simulink model "pendulum3D_nonlinear_control_cascade_simulation"  (R2017a)
settings: Solver=FixedStepAuto  StartTime=0.0  StopTime=30  FixedStep=dt  RelTol=1e-3
values from neighbouring files (symbols this model uses):
  d_x = 7    [simulation_initalization.m]
  d_y = 4    [simulation_initalization.m]
  dt = 1e-3    (= 0.001)    [f_simulink3d.m]    (also in simulation_initalization.m)
  Kdx_t = 3.324    [simulation_initalization.m]
  Kdy_t = 0.4079    [simulation_initalization.m]
  Kix = 0.103    [simulation_initalization.m]
  Kiy = 0.07209    [simulation_initalization.m]
  Kpx = 0.577    [simulation_initalization.m]
  Kpx_t = 4.786    [simulation_initalization.m]
  Kpy = 0.7879    [simulation_initalization.m]
  Kpy_t = 1.002    [simulation_initalization.m]
  L = 2.0    (= 2)    [compensator_phix.m]    (also in compensator_phiy.m; f_simulink3d.m; pendulum_dynamics.m; simulation_initalization.m)
  phi_init = [phix_init, phiy_init]    [simulation_initalization.m]
  pt_init = [x_init, y_init, z_init]    [simulation_initalization.m]
  x_init = 2.6192    [simulation_initalization.m]
  y_init = 0    [simulation_initalization.m]
  z_init = 2.24    [simulation_initalization.m]
libraries: simulink x4, sharedTrackingLibrary x1
settings Model: Creator=Workstation  LastModifiedBy=Jan

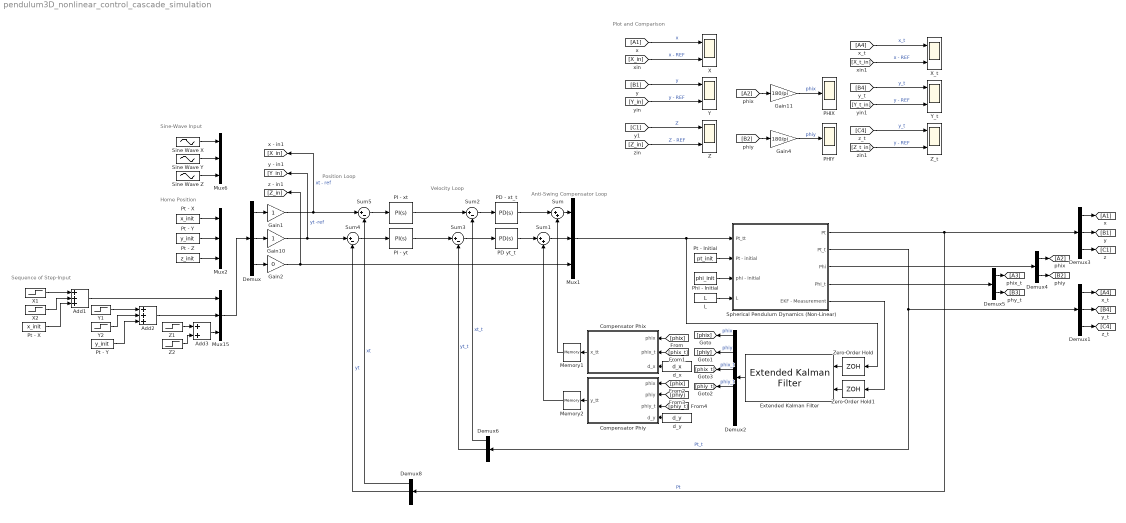
== system pendulum3D_nonlinear_control_cascade_simulation ==
  note: Sequence of Step-Input
  note: Home Position
  note: Sine-Wave Input
  note: Position Loop
  note: Velocity Loop
  note: Anti-Swing Compensator Loop
  note: Plot and Comparison
  Add1 : Sum  Inputs=+++
  Add2 : Sum  Inputs=+++
  Add3 : Sum
  Compensator Phix : MATLAB Function  TreatAsAtomicUnit=on
  Compensator Phiy : MATLAB Function  TreatAsAtomicUnit=on
  Demux{,1,3,6,8} (5 alike) : Demux  Outputs=3
  Demux2 : Demux  Outputs=6
  Demux4 : Demux  Outputs=2
  Demux5 : Demux  Outputs=2
  Extended Kalman Filter : sharedTrackingLibrary/Extended Kalman Filter  StateTransitionFcn=f_simulink3d  HasStateTransitionJacobianFcn=off  HasAdditiveProcessNoise=Additive  ProcessNoise=Q  HasTimeVaryingProcessNoise=off  HasStateTransitionFcnExtraArgument=1  InitialState=zeros(6,1)  InitialStateCovariance=P  MeasurementFcn1=h_simulink3d  HasMeasurementJacobianFcn1=off  HasMeasurementEnablePort1=off  HasAdditiveMeasurementNoise1=Additive  MeasurementNoise1=R  HasTimeVaryingMeasurementNoise1=off  HasMeasurementFcnExtraArgument1=0  MeasurementFcn2=myMeasurementFcn  HasMeasurementJacobianFcn2=off  HasMeasurementEnablePort2=off  HasAdditiveMeasurementNoise2=Additive  MeasurementNoise2=1  HasTimeVaryingMeasurementNoise2=off  HasMeasurementFcnExtraArgument2=0  MeasurementFcn3=myMeasurementFcn  HasMeasurementJacobianFcn3=off  HasMeasurementEnablePort3=off  HasAdditiveMeasurementNoise3=Additive  MeasurementNoise3=1  HasTimeVaryingMeasurementNoise3=off  HasMeasurementFcnExtraArgument3=0  MeasurementFcn4=myMeasurementFcn  HasMeasurementJacobianFcn4=off  HasMeasurementEnablePort4=off  HasAdditiveMeasurementNoise4=Additive  MeasurementNoise4=1  HasTimeVaryingMeasurementNoise4=off  HasMeasurementFcnExtraArgument4=0  MeasurementFcn5=myMeasurementFcn  HasMeasurementJacobianFcn5=off  HasMeasurementEnablePort5=off  HasAdditiveMeasurementNoise5=Additive  MeasurementNoise5=1  HasTimeVaryingMeasurementNoise5=off  HasMeasurementFcnExtraArgument5=0  EnableMultirate=off  StateTransitionFcnSampleTime=1  MeasurementFcn1SampleTime=1  MeasurementFcn2SampleTime=1  MeasurementFcn3SampleTime=1  MeasurementFcn4SampleTime=1  MeasurementFcn5SampleTime=1  UseCurrentEstimator=on  OutputStateCovariance=off  DataType=double  SampleTime=dt  NumberOfMeasurements=1
  Gain1 : Gain
  Gain10 : Gain
  Gain11 : Gain  Gain=180/pi
  Gain2 : Gain  Gain=0
  Gain4 : Gain  Gain=180/pi
  L : Constant  Value=L
  Memory1 : Memory
  Memory2 : Memory
  Mux{1..2,6,15} (4 alike) : Mux  Inputs=3
  PD - xt_t : simulink/Continuous/PID Controller  Controller=PD  TimeDomain=Continuous-time  SampleTime=-1  IntegratorMethod=Forward Euler  FilterMethod=Forward Euler  Form=Parallel  UseFilter=on  ControllerParametersSource=internal  P=Kpx_t  I=1  D=Kdx_t  N=100  InitialConditionSource=internal  InitialConditionForIntegrator=0  InitialConditionForFilter=0  ExternalReset=none  LimitOutput=off  UpperSaturationLimit=inf  LowerSaturationLimit=-inf  LinearizeAsGain=on  AntiWindupMode=none  Kb=1  TrackingMode=off  Kt=1  PParamMin=[]  PParamMax=[]  IParamMin=[]  IParamMax=[]  DParamMin=[]  DParamMax=[]  NParamMin=[]  NParamMax=[]  KbParamMin=[]  KbParamMax=[]  KtParamMin=[]  KtParamMax=[]  POutMin=[]  POutMax=[]  IOutMin=[]  IOutMax=[]  DOutMin=[]  DOutMax=[]  NOutMin=[]  NOutMax=[]  KbOutMin=[]  KbOutMax=[]  KtOutMin=[]  KtOutMax=[]  IntegratorOutMin=[]  IntegratorOutMax=[]  FilterOutMin=[]  FilterOutMax=[]  SumOutMin=[]  SumOutMax=[]  SumI1OutMin=[]  SumI1OutMax=[]  SumI2OutMin=[]  SumI2OutMax=[]  SumI3OutMin=[]  SumI3OutMax=[]  SumDOutMin=[]  SumDOutMax=[]  SaturationOutMin=[]  SaturationOutMax=[]  IntegratorContinuousStateAttributes=''  IntegratorStateMustResolveToSignalObject=off  IntegratorRTWStateStorageClass=Auto  FilterContinuousStateAttributes=''  FilterStateMustResolveToSignalObject=off  FilterRTWStateStorageClass=Auto  DifferentiatorICPrevScaledInput=0  DifferentiatorOutMin=[]  DifferentiatorOutMax=[]  InitialConditionSetting=State (most efficient)
  PD yt_t : simulink/Continuous/PID Controller  Controller=PD  TimeDomain=Continuous-time  SampleTime=-1  IntegratorMethod=Forward Euler  FilterMethod=Forward Euler  Form=Parallel  UseFilter=on  ControllerParametersSource=internal  P=Kpy_t  I=1  D=Kdy_t  N=100  InitialConditionSource=internal  InitialConditionForIntegrator=0  InitialConditionForFilter=0  ExternalReset=none  LimitOutput=off  UpperSaturationLimit=inf  LowerSaturationLimit=-inf  LinearizeAsGain=on  AntiWindupMode=none  Kb=1  TrackingMode=off  Kt=1  PParamMin=[]  PParamMax=[]  IParamMin=[]  IParamMax=[]  DParamMin=[]  DParamMax=[]  NParamMin=[]  NParamMax=[]  KbParamMin=[]  KbParamMax=[]  KtParamMin=[]  KtParamMax=[]  POutMin=[]  POutMax=[]  IOutMin=[]  IOutMax=[]  DOutMin=[]  DOutMax=[]  NOutMin=[]  NOutMax=[]  KbOutMin=[]  KbOutMax=[]  KtOutMin=[]  KtOutMax=[]  IntegratorOutMin=[]  IntegratorOutMax=[]  FilterOutMin=[]  FilterOutMax=[]  SumOutMin=[]  SumOutMax=[]  SumI1OutMin=[]  SumI1OutMax=[]  SumI2OutMin=[]  SumI2OutMax=[]  SumI3OutMin=[]  SumI3OutMax=[]  SumDOutMin=[]  SumDOutMax=[]  SaturationOutMin=[]  SaturationOutMax=[]  IntegratorContinuousStateAttributes=''  IntegratorStateMustResolveToSignalObject=off  IntegratorRTWStateStorageClass=Auto  FilterContinuousStateAttributes=''  FilterStateMustResolveToSignalObject=off  FilterRTWStateStorageClass=Auto  DifferentiatorICPrevScaledInput=0  DifferentiatorOutMin=[]  DifferentiatorOutMax=[]  InitialConditionSetting=State (most efficient)
  PHIX : Scope
  PHIY : Scope
  PI - xt : simulink/Continuous/PID Controller  Controller=PI  TimeDomain=Continuous-time  SampleTime=-1  IntegratorMethod=Forward Euler  FilterMethod=Forward Euler  Form=Parallel  UseFilter=on  ControllerParametersSource=internal  P=Kpx  I=Kix  D=Kix  N=100  InitialConditionSource=internal  InitialConditionForIntegrator=0  InitialConditionForFilter=0  ExternalReset=none  LimitOutput=off  UpperSaturationLimit=inf  LowerSaturationLimit=-inf  LinearizeAsGain=on  AntiWindupMode=none  Kb=1  TrackingMode=off  Kt=1  PParamMin=[]  PParamMax=[]  IParamMin=[]  IParamMax=[]  DParamMin=[]  DParamMax=[]  NParamMin=[]  NParamMax=[]  KbParamMin=[]  KbParamMax=[]  KtParamMin=[]  KtParamMax=[]  POutMin=[]  POutMax=[]  IOutMin=[]  IOutMax=[]  DOutMin=[]  DOutMax=[]  NOutMin=[]  NOutMax=[]  KbOutMin=[]  KbOutMax=[]  KtOutMin=[]  KtOutMax=[]  IntegratorOutMin=[]  IntegratorOutMax=[]  FilterOutMin=[]  FilterOutMax=[]  SumOutMin=[]  SumOutMax=[]  SumI1OutMin=[]  SumI1OutMax=[]  SumI2OutMin=[]  SumI2OutMax=[]  SumI3OutMin=[]  SumI3OutMax=[]  SumDOutMin=[]  SumDOutMax=[]  SaturationOutMin=[]  SaturationOutMax=[]  IntegratorContinuousStateAttributes=''  IntegratorStateMustResolveToSignalObject=off  IntegratorRTWStateStorageClass=Auto  FilterContinuousStateAttributes=''  FilterStateMustResolveToSignalObject=off  FilterRTWStateStorageClass=Auto  DifferentiatorICPrevScaledInput=0  DifferentiatorOutMin=[]  DifferentiatorOutMax=[]  InitialConditionSetting=State (most efficient)
  PI - yt : simulink/Continuous/PID Controller  Controller=PI  TimeDomain=Continuous-time  SampleTime=-1  IntegratorMethod=Forward Euler  FilterMethod=Forward Euler  Form=Parallel  UseFilter=on  ControllerParametersSource=internal  P=Kpy  I=Kiy  D=0  N=100  InitialConditionSource=internal  InitialConditionForIntegrator=0  InitialConditionForFilter=0  ExternalReset=none  LimitOutput=off  UpperSaturationLimit=inf  LowerSaturationLimit=-inf  LinearizeAsGain=on  AntiWindupMode=none  Kb=1  TrackingMode=off  Kt=1  PParamMin=[]  PParamMax=[]  IParamMin=[]  IParamMax=[]  DParamMin=[]  DParamMax=[]  NParamMin=[]  NParamMax=[]  KbParamMin=[]  KbParamMax=[]  KtParamMin=[]  KtParamMax=[]  POutMin=[]  POutMax=[]  IOutMin=[]  IOutMax=[]  DOutMin=[]  DOutMax=[]  NOutMin=[]  NOutMax=[]  KbOutMin=[]  KbOutMax=[]  KtOutMin=[]  KtOutMax=[]  IntegratorOutMin=[]  IntegratorOutMax=[]  FilterOutMin=[]  FilterOutMax=[]  SumOutMin=[]  SumOutMax=[]  SumI1OutMin=[]  SumI1OutMax=[]  SumI2OutMin=[]  SumI2OutMax=[]  SumI3OutMin=[]  SumI3OutMax=[]  SumDOutMin=[]  SumDOutMax=[]  SaturationOutMin=[]  SaturationOutMax=[]  IntegratorContinuousStateAttributes=''  IntegratorStateMustResolveToSignalObject=off  IntegratorRTWStateStorageClass=Auto  FilterContinuousStateAttributes=''  FilterStateMustResolveToSignalObject=off  FilterRTWStateStorageClass=Auto  DifferentiatorICPrevScaledInput=0  DifferentiatorOutMin=[]  DifferentiatorOutMax=[]  InitialConditionSetting=State (most efficient)
  Phi - Initial : Constant  Value=phi_init
  Pt - Initial : Constant  Value=pt_init
  Pt - X : Constant  Value=x_init
  "Pt - X " : Constant  Value=x_init
  Pt - Y : Constant  Value=y_init
  "Pt - Y " : Constant  Value=y_init
  Pt - Z : Constant  Value=z_init
  Sine Wave X : Sin  Amplitude=0.5  Bias=x_init  Frequency=2*pi*0.07  SampleTime=0
  Sine Wave Y : Sin  Amplitude=0.3  Bias=y_init  Frequency=2*pi*0.09  SampleTime=0
  Sine Wave Z : Sin  Amplitude=0.25  Bias=z_init  Frequency=2*pi*0.15  SampleTime=0
  Spherical Pendulum Dynamics (Non-Linear) : Subsystem
  Sum : Sum  Inputs=|++
  Sum1 : Sum  Inputs=|++
  Sum{2..5} (4 alike) : Sum  Inputs=|+-
  X : Scope  NumInputPorts=2
  X1 : Step  After=0.4  SampleTime=0
  X2 : Step  Time=10  After=-0.8  SampleTime=0
  X_t : Scope  NumInputPorts=2
  Y : Scope  NumInputPorts=2
  Y1 : Step  Time=2  After=0.4  SampleTime=0
  Y2 : Step  Time=13  After=-0.8  SampleTime=0
  Y_t : Scope  NumInputPorts=2
  Z : Scope  NumInputPorts=2
  Z1 : Step  Time=3  After=0.4  SampleTime=0
  Z2 : Step  Time=9  After=-0.2  SampleTime=0
  Z_t : Scope  NumInputPorts=2
  Zero-Order Hold : ZeroOrderHold  SampleTime=dt
  Zero-Order Hold1 : ZeroOrderHold  SampleTime=dt
  d_x : Constant  Value=d_x
  d_y : Constant  Value=d_y
  wires:
  Zero-Order Hold/1 -> Extended Kalman Filter/1
  Zero-Order Hold1/1 -> Extended Kalman Filter/2
  Spherical Pendulum Dynamics (Non-Linear)/5(EKF - Measurement) -> Zero-Order Hold1/1
  Extended Kalman Filter/1 -> Demux2/1
  Sum1/1 -> Mux1/2
  PD - xt_t/1 -> Sum/1
  Sum/1 -> Mux1/1
  Mux1/1 -> Zero-Order Hold/1, Spherical Pendulum Dynamics (Non-Linear)/1(Pt_tt)
  Pt - Initial/1 -> Spherical Pendulum Dynamics (Non-Linear)/2(Pt - initial)
  Phi - Initial/1 -> Spherical Pendulum Dynamics (Non-Linear)/3(phi - initial)
  Demux5/1 -> [A3]
  Spherical Pendulum Dynamics (Non-Linear)/3(Phi) -> Demux4/1
  Demux5/2 -> [B3]
  Demux4/2 -> [B2]
  Spherical Pendulum Dynamics (Non-Linear)/4(Phi_t) -> Demux5/1
  Demux4/1 -> [A2]
  Demux3/2 -> [B1]
  Demux3/1 -> [A1]
  Spherical Pendulum Dynamics (Non-Linear)/1(Pt) -> Demux8/1, Demux3/1  "Pt"
  Demux3/3 -> [C1]
  Demux1/2 -> [B4]
  Demux1/3 -> [C4]
  [C1] -> Z/1  "Z"
  [Y_in] -> Y/2  "y - REF"
  [Z_in] -> Z/2  "Z - REF"
  Gain11/1 -> PHIX/1  "phix"
  [B2] -> Gain4/1
  Gain4/1 -> PHIY/1  "phiy"
  [A1] -> X/1  "x"
  [B1] -> Y/1  "y"
  [A2] -> Gain11/1
  [X_in] -> X/2  "x - REF"
  [B4] -> Y_t/1  "y_t"
  [A4] -> X_t/1  "x_t"
  [Z_t_in] -> Z_t/2  "y - REF"
  [X_t_in] -> X_t/2  "x - REF"
  [Y_t_in] -> Y_t/2  "y - REF"
  [C4] -> Z_t/1  "y_t"
  Sum2/1 -> PD - xt_t/1
  PD yt_t/1 -> Sum1/1
  Sum4/1 -> PI - yt/1
  Sum5/1 -> PI - xt/1
  Sum3/1 -> PD yt_t/1
  Demux6/1 -> Sum2/2  "xt_t"
  Demux6/2 -> Sum3/2  "yt_t"
  Spherical Pendulum Dynamics (Non-Linear)/2(Pt_t) -> Demux6/1, Demux1/1  "Pt_t"
  Demux1/1 -> [A4]
  Gain1/1 -> Sum5/1, [X_in]  "xt - ref"
  Gain10/1 -> Sum4/1, [Y_in]  "yt -ref"
  Demux8/1 -> Sum5/2  "xt"
  Demux8/2 -> Sum4/2  "yt"
  Add2/1 -> Mux15/2
  Add1/1 -> Mux15/1
  PI - xt/1 -> Sum2/1
  PI - yt/1 -> Sum3/1
  d_x/1 -> Compensator Phix/3(d_x)
  Compensator Phix/1(x_tt) -> Memory1/1
  [phix] -> Compensator Phix/1(phix)
  [phix_t] -> Compensator Phix/2(phix_t)
  d_y/1 -> Compensator Phiy/4(d_y)
  [phiy_t] -> Compensator Phiy/3(phiy_t)
  [phiy] -> Compensator Phiy/2(phiy)
  [phix] -> Compensator Phiy/1(phix)
  Compensator Phiy/1(y_tt) -> Memory2/1
  Memory2/1 -> Sum1/2
  Memory1/1 -> Sum/2
  Demux2/1 -> [phix]  "phix"
  Demux2/2 -> [phiy]  "phiy"
  Demux2/4 -> [phiy_t]  "phiy_t"
  Demux2/3 -> [phix_t]  "phix_t"
  Gain2/1 -> Mux1/3, [Z_in]
  Z2/1 -> Add3/2
  Y2/1 -> Add2/2
  Z1/1 -> Add3/1
  X2/1 -> Add1/2
  Y1/1 -> Add2/1
  Demux/3 -> Gain2/1
  X1/1 -> Add1/1
  Pt - X/1 -> Add1/3
  "Pt - Y "/1 -> Add2/3
  Demux/2 -> Gain10/1
  Demux/1 -> Gain1/1
  Pt - Y/1 -> Mux2/2
  Pt - Z/1 -> Mux2/3
  Sine Wave X/1 -> Mux6/1
  Sine Wave Y/1 -> Mux6/2
  Sine Wave Z/1 -> Mux6/3
  "Pt - X "/1 -> Mux2/1
  Add3/1 -> Mux15/3
  L/1 -> Spherical Pendulum Dynamics (Non-Linear)/4(L)
  Mux15/1 -> Demux/1

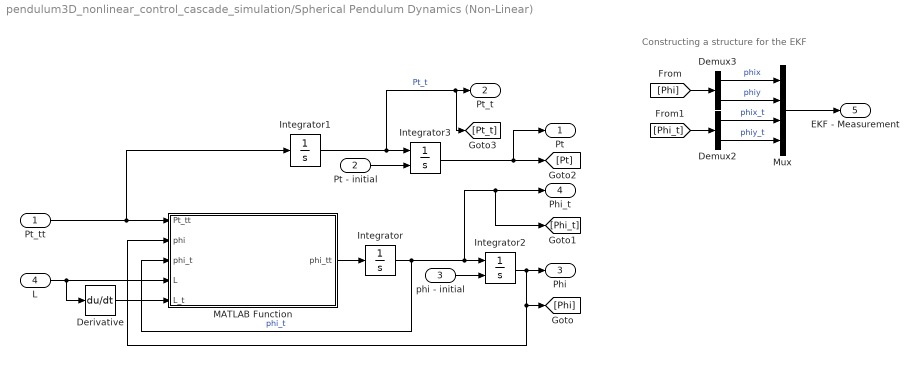
== system pendulum3D_nonlinear_control_cascade_simulation/Spherical Pendulum Dynamics (Non-Linear) ==
  note: Constructing a structure
      | for the EKF
  Pt_tt : Inport
  Pt - initial : Inport  Port=2
  phi - initial : Inport  Port=3
  L : Inport  Port=4
  Demux2 : Demux  Outputs=2
  Demux3 : Demux  Outputs=2
  Derivative : Derivative
  Integrator : Integrator  InitialCondition=[0 0]
  Integrator1 : Integrator  InitialCondition=[0 0 0]
  Integrator2 : Integrator  InitialConditionSource=external
  Integrator3 : Integrator  InitialConditionSource=external
  MATLAB Function : MATLAB Function  TreatAsAtomicUnit=on
  Mux : Mux
  Pt : Outport
  Pt_t : Outport  Port=2
  Phi : Outport  Port=3
  Phi_t : Outport  Port=4
  EKF - Measurement : Outport  Port=5
  wires:
  Integrator2/1 -> [Phi], MATLAB Function/2(phi), Phi/1
  Integrator3/1 -> Pt/1, [Pt]
  Integrator/1 -> MATLAB Function/3(phi_t), Integrator2/1, [Phi_t], Phi_t/1  "phi_t"
  Pt - initial/1 -> Integrator3/2
  phi - initial/1 -> Integrator2/2
  Pt_tt/1 -> MATLAB Function/1(Pt_tt), Integrator1/1
  MATLAB Function/1(phi_tt) -> Integrator/1
  Integrator1/1 -> [Pt_t], Pt_t/1, Integrator3/1  "Pt_t"
  [Phi_t] -> Demux2/1
  [Phi] -> Demux3/1
  Demux2/1 -> Mux/3  "phix_t"
  Demux2/2 -> Mux/4  "phiy_t"
  Mux/1 -> EKF - Measurement/1
  Demux3/1 -> Mux/1  "phix"
  Demux3/2 -> Mux/2  "phiy"
  L/1 -> MATLAB Function/4(L), Derivative/1
  Derivative/1 -> MATLAB Function/5(L_t)

== matlab function pendulum3D_nonlinear_control_cascade_simulation/Spherical Pendulum Dynamics (Non-Linear)/MATLAB Function ==
  data: Pt_tt input; phi input; phi_tt output; phi_t input; L input; L_t input
function phi_tt = pendulum_dynamics(Pt_tt, phi, phi_t,L,L_t)
    
    g = 9.81;   % Gravity
%     L = 2.0;    % Wire length
%     L_t = 0;    % Constant wire length
    
    % Tool-point acceleration components
    xt_tt = Pt_tt(1); 
    yt_tt = Pt_tt(2); 
    zt_tt = Pt_tt(3);

    % Pendulum euler angles (angular position)
    phix = phi(1);
    phiy = phi(2);

    % Pendulum euler angles (angular velocity)
    phix_t = phi_t(1);
    phiy_t = phi_t(2);
    
     % Pendulum ODE of the euler angles
    % (found from euler-lagrange equation,
    %  derived by the use of Maple)
    phix_tt = (xt_tt*cos(phix) + yt_tt*sin(phix)*sin(phiy) ...
              - zt_tt*sin(phix)*cos(phiy) ...
              - g*sin(phix)*cos(phiy) ...
              - 2*L_t*phix_t ...
              - L*phiy_t^2*sin(phix)*cos(phix)) / L;

    phiy_tt = (- yt_tt*cos(phiy) - zt_tt*sin(phiy) ...
              - g*sin(phiy) + 2*L_t*phiy_t*cos(phix) ...
              + 2*L*phix_t*phiy_t*sin(phix)) ...
              / (L*cos(phix));

    phi_tt = [phix_tt; phiy_tt];

== matlab function pendulum3D_nonlinear_control_cascade_simulation/Compensator Phiy ==
  data: phix input; phiy input; y_tt output; phiy_t input; d_y input
function y_tt = compensator_phiy(phix, phiy, phiy_t, d_y)
    % Constants
    L = 2.0;  % Wire Length
   
    y_tt = L*d_y*phiy_t*cos(phix) /cos(phiy);

== matlab function pendulum3D_nonlinear_control_cascade_simulation/Compensator Phix ==
  data: phix input; x_tt output; phix_t input; d_x input
function x_tt = compensator_phix(phix, phix_t, d_x)
    % Constants
    L = 2.0;  % Wire Length
    
    x_tt = -L*d_x*phix_t /cos(phix);
